simulink model "pendulum"  (Simulink 8.6)
settings: Solver=ode45  StartTime=0.0  StopTime=20  RelTol=1e-3
settings Model: Creator=jmavisser  LastModifiedBy=winfredmugge
settings OptimizationCC: InitFltsAndDblsToZero=on
settings DebuggingCC: SaveWithParameterizedLinksMsg=none  SignalResolutionControl=TryResolveAllWithWarning  MultiTaskDSMMsg=warning  MultiTaskCondExecSysMsg=none  FcnCallInpInsideContextMsg=UseLocalSettings
settings GRTTargetCC: TargetFcnLib=ansi_tfl_tmw.mat
settings ConfigComp: CovSFcnEnable=off

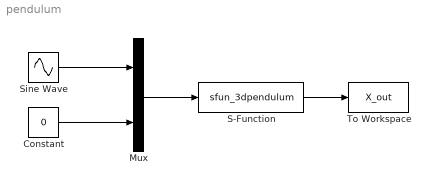
== system pendulum ==
  Constant : Constant  Value=0
  Mux : Mux  Inputs=2
  S-Function : S-Function  FunctionName=sfun_3dpendulum  SFunctionDeploymentMode=off  EnableBusSupport=off
  Sine Wave : Sin  Amplitude=3  SampleTime=0
  To Workspace : ToWorkspace  VariableName=X_out  SaveFormat=Structure With Time  SampleTime=0.05
  wires:
  S-Function/1 -> To Workspace/1
  Mux/1 -> S-Function/1
  Constant/1 -> Mux/2
  Sine Wave/1 -> Mux/1
